simulink model "robot3_model_mob_control2"  (R2023b)
settings: Solver=FixedStepAuto  StartTime=0.0  StopTime=2*pi  RelTol=1e-3
undefined symbols (not defined in the file or in its folder): Cartesian_trajectory, Coriolis3, CoriolisT3, Dhat3, Dinv3, Forward_kin3, Gravity3, Ko3
libraries: simulink x1
settings Model: Creator=사용자  LastModifiedBy=rodel
settings SolverCC: ZeroCrossAlgorithm=Adaptive
settings DebuggingCC: IgnoredZcDiagnostic=none

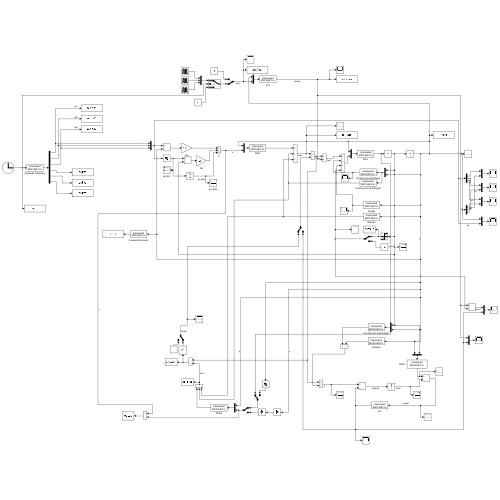
[thumbnail: Simulink's stored preview of the top-level diagram]
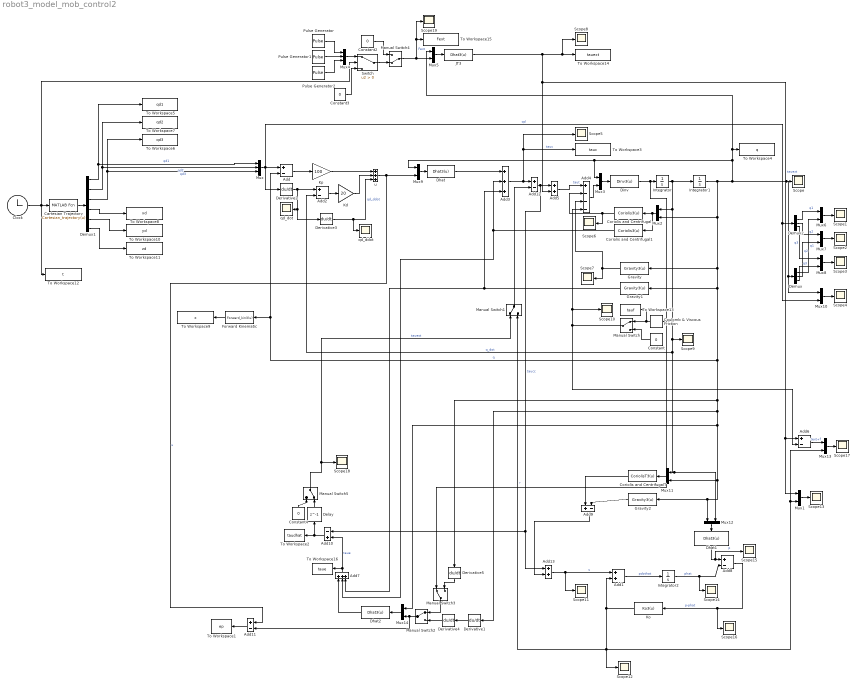
== system robot3_model_mob_control2 ==
  Add{,2,6,8..9,11..12} (7 alike) : Sum  Inputs=+-
  Add1 : Sum
  Add10 : Sum  Inputs=-+
  Add13 : Sum
  Add3 : Sum  Inputs=+++
  Add4 : Sum  Inputs=+---
  Add5 : Sum
  Add7 : Sum  Inputs=+++
  Cartesian Trajectory : MATLABFcn  MATLABFcn=Cartesian_trajectory(u)  OutputDimensions=6  Output1D=off
  Clock : Clock
  Constant{,2..4} (4 alike) : Constant  Value=0
  Coriolis and Centrifugal : MATLABFcn  MATLABFcn=Coriolis3(u)  OutputDimensions=3  Output1D=off
  Coriolis and Centrifugal1 : MATLABFcn  MATLABFcn=Coriolis3(u)  OutputDimensions=3  Output1D=off
  Coriolis and CentrifugalT : MATLABFcn  MATLABFcn=CoriolisT3(u)  OutputDimensions=3  Output1D=off
  Coulomb & Viscous Friction : simulink/Discontinuities/Coulomb & Viscous Friction  offset=5  gain=3
  Delay : Delay  DelayLength=1  InitialCondition=0
  Demux : Demux  Outputs=3
  Demux1 : Demux  Outputs=6
  Demux2 : Demux  Outputs=3
  Derivative{1..5} (5 alike) : Derivative
  Dhat : MATLABFcn  MATLABFcn=Dhat3(u)  OutputDimensions=3  Output1D=off
  Dhat1 : MATLABFcn  MATLABFcn=Dhat3(u)  OutputDimensions=3  Output1D=off
  Dhat2 : MATLABFcn  MATLABFcn=Dhat3(u)  OutputDimensions=3  Output1D=off
  Dinv : MATLABFcn  MATLABFcn=Dinv3(u)  OutputDimensions=3  Output1D=off
  Forward Kinematic : MATLABFcn  MATLABFcn=Forward_kin3(u)  OutputDimensions=3  Output1D=off
  Gravity : MATLABFcn  MATLABFcn=Gravity3(u)  OutputDimensions=3  Output1D=off
  Gravity1 : MATLABFcn  MATLABFcn=Gravity3(u)  OutputDimensions=3  Output1D=off
  Gravity2 : MATLABFcn  MATLABFcn=Gravity3(u)  OutputDimensions=3  Output1D=off
  Integrator : Integrator  InitialCondition=[0;0;0];
  Integrator1 : Integrator  InitialCondition=[0.9587;0.7246;-1.1694]
  Integrator2 : Integrator  InitialCondition=[0;0;0];
  JT3 : MATLABFcn  MATLABFcn=Dhat3(u)  OutputDimensions=3  Output1D=off
  Kd : Gain  Gain=20
  Ko : MATLABFcn  MATLABFcn=Ko3(u)  OutputDimensions=3  Output1D=off
  Kp : Gain  Gain=100
  Manual Switch{,1..3} (4 alike) : ManualSwitch
  Manual Switch4 : ManualSwitch  CurrentSetting=0
  Manual Switch5 : ManualSwitch  CurrentSetting=0
  Mux : Mux  Inputs=3
  Mux{1..3,5..14} (13 alike) : Mux  Inputs=2
  Mux4 : Mux  Inputs=3
  Pulse Generator : DiscretePulseGenerator  PulseType=Time based  Amplitude=10  PulseWidth=2  PhaseDelay=2
  Pulse Generator1 : DiscretePulseGenerator  PulseType=Time based  Amplitude=10  PhaseDelay=3
  Pulse Generator2 : DiscretePulseGenerator  PulseType=Time based  Amplitude=30  PulseWidth=20  PhaseDelay=1
  Scope{,1..19} (20 alike) : Scope
  Switch : Switch  Criteria=u2 > Threshold  SaturateOnIntegerOverflow=off  InputSameDT=off
  To Workspace1 : ToWorkspace  VariableName=ep  SaveFormat=Timeseries  SampleTime=0.001
  To Workspace10 : ToWorkspace  VariableName=yd  SampleTime=0.001
  To Workspace11 : ToWorkspace  VariableName=zd  SampleTime=0.001
  To Workspace12 : ToWorkspace  VariableName=t  SaveFormat=Timeseries  SampleTime=0.001
  To Workspace13 : ToWorkspace  VariableName=tauf  SaveFormat=Timeseries  SampleTime=0.001
  To Workspace14 : ToWorkspace  VariableName=tauext  SaveFormat=Timeseries  SampleTime=0.001
  To Workspace15 : ToWorkspace  VariableName=Fext  SaveFormat=Timeseries  SampleTime=0.001
  To Workspace16 : ToWorkspace  VariableName=taue  SaveFormat=Timeseries  SampleTime=0.001
  To Workspace2 : ToWorkspace  VariableName=taudhat  SaveFormat=Timeseries  SampleTime=0.001
  To Workspace3 : ToWorkspace  VariableName=tauc  SaveFormat=Timeseries  SampleTime=0.001
  To Workspace4 : ToWorkspace  VariableName=q  SaveFormat=Timeseries  SampleTime=0.001
  To Workspace5 : ToWorkspace  VariableName=qd1  SaveFormat=Timeseries  SampleTime=0.001
  To Workspace6 : ToWorkspace  VariableName=qd3  SaveFormat=Timeseries  SampleTime=0.001
  To Workspace7 : ToWorkspace  VariableName=qd2  SaveFormat=Timeseries  SampleTime=0.001
  To Workspace8 : ToWorkspace  VariableName=xd  SampleTime=0.001
  To Workspace9 : ToWorkspace  VariableName=x  SampleTime=0.001
  qd_ddot : Scope
  qd_dot : Scope
  u : Sum  Inputs=+++
  wires:
  Mux/1 -> Derivative2/1, Mux10/2, Demux2/1, Add/1  "qd"
  Add2/1 -> Kd/1
  Kp/1 -> u/1
  Kd/1 -> u/2
  Add/1 -> Kp/1
  Mux2/1 -> Coriolis and Centrifugal/1, Coriolis and Centrifugal1/1
  Integrator/1 -> Mux12/2, Mux11/1, Add2/2, Scope9/1, Coulomb & Viscous Friction/1, Mux2/1, Integrator1/1  "q_dot"
  Derivative3/1 -> qd_ddot/1, u/3  "qd_ddot"
  Mux9/1 -> Dhat/1
  Mux3/1 -> Dinv/1
  Dhat/1 -> Add3/1
  Coriolis and Centrifugal/1 -> Add4/2, Scope6/1
  Gravity/1 -> Add4/3, Scope7/1
  Constant/1 -> Manual Switch/2
  Coulomb & Viscous Friction/1 -> To Workspace13/1, Manual Switch/1
  Derivative2/1 -> Derivative3/1, qd_dot/1, Add2/1
  Forward Kinematic/1 -> To Workspace9/1
  Demux1/5 -> To Workspace10/1
  Demux1/4 -> To Workspace8/1
  Demux1/3 -> To Workspace6/1, Mux/3  "qd3"
  Cartesian Trajectory/1 -> Demux1/1
  Demux1/1 -> To Workspace5/1, Mux/1  "qd1"
  Clock/1 -> Switch/2, Cartesian Trajectory/1, To Workspace12/1
  Demux1/6 -> To Workspace11/1
  Demux1/2 -> Mux/2, To Workspace7/1  "qd2"
  Add3/1 -> Scope5/1, To Workspace3/1, Add12/1  "tauc"
  Pulse Generator/1 -> Mux4/1
  Pulse Generator1/1 -> Mux4/2
  Pulse Generator2/1 -> Mux4/3
  Mux4/1 -> Switch/1
  Constant3/1 -> Switch/3
  Switch/1 -> Manual Switch4/2
  Constant2/1 -> Manual Switch4/1
  Demux/2 -> Mux7/2  "q2"
  Mux6/1 -> Scope1/1
  Mux7/1 -> Scope2/1
  Mux8/1 -> Scope3/1
  Demux/1 -> Mux6/2  "q1"
  Demux/3 -> Mux8/2  "q3"
  Mux10/1 -> Scope4/1
  Demux2/1 -> Mux6/1  "q1"
  Demux2/2 -> Mux7/1  "q2"
  Demux2/3 -> Mux8/1  "q3"
  Gravity2/1 -> Add9/2
  Mux11/1 -> Coriolis and CentrifugalT/1
  Add9/1 -> Add13/2
  Add4/1 -> Mux3/2
  Coriolis and CentrifugalT/1 -> Add9/1
  Add5/1 -> Add4/1  "taut"
  Manual Switch/1 -> Add6/2, Scope10/1, Add4/4
  JT3/1 -> Add6/1, Mux1/1, Add5/2, To Workspace14/1, Scope8/1  "tauext"
  Manual Switch4/1 -> Scope19/1, To Workspace15/1, Mux5/2  "Fext"
  Mux5/1 -> JT3/1
  Add13/1 -> Scope11/1, Add1/1  "u"
  Add1/1 -> Integrator2/1  "pdothat"
  Integrator2/1 -> Scope14/1, Add8/2  "phat"
  Add8/1 -> Scope16/1, Ko/1  "p-phat"
  Ko/1 -> Scope12/1, Mux1/2, Mux13/2, Manual Switch1/2, Add1/2  "r"
  Dhat1/1 -> Scope15/1, Add8/1  "p"
  Mux12/1 -> Dhat1/1
  Mux1/1 -> Scope13/1
  Add6/1 -> Mux13/1  "text+f"
  Mux13/1 -> Scope17/1
  Mux14/1 -> Dhat2/1
  Derivative1/1 -> Derivative4/1
  Manual Switch2/1 -> Add11/2, Mux14/2
  Coriolis and Centrifugal1/1 -> Add7/2, Add3/2
  Integrator1/1 -> Mux10/1, Demux/1, Scope/1, Mux3/1, Mux9/1, Mux5/1, To Workspace4/1, Mux2/2, Forward Kinematic/1, Add/2, Mux12/1, Gravity2/1, Mux11/2, Mux14/1, Derivative1/1, Derivative5/1, Gravity1/1, Gravity/1  "q"
  Manual Switch3/1 -> Manual Switch2/1
  Derivative4/1 -> Manual Switch2/2
  Derivative5/1 -> Manual Switch3/2
  u/1 -> Mux9/2, Add11/1  "u"
  Add7/1 -> To Workspace16/1, Add10/2  "taue"
  Gravity1/1 -> Add7/3, Add3/3
  Dhat2/1 -> Add7/1
  Add11/1 -> To Workspace1/1
  Add10/1 -> Delay/1, To Workspace2/1
  Delay/1 -> Manual Switch5/2
  Constant4/1 -> Manual Switch5/1
  Manual Switch5/1 -> Manual Switch1/1, Scope18/1  "tauest"
  Add12/1 -> Add5/1, Add10/1, Add13/1  "taucc"
  Dinv/1 -> Manual Switch3/1, Integrator/1
  Manual Switch1/1 -> Add12/2
